simulink model "Measure_BH_curve1"  (R2014a)
settings: Solver=ode23tb  StartTime=0.0  StopTime=0.08  RelTol=1e-3
libraries: powerlib x9, simulink x1
settings Model: Creator=Administrator  LastModifiedBy=Administrator

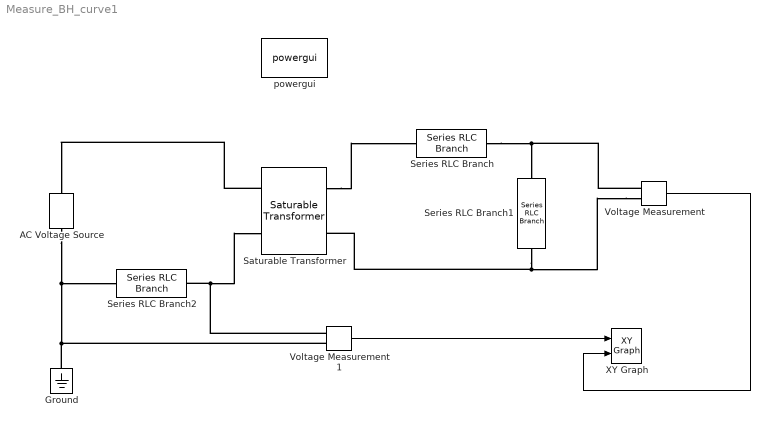
== system Measure_BH_curve1 ==
  AC Voltage Source : powerlib/Electrical Sources/AC Voltage Source  Amplitude=10e5*sqrt(2)  Phase=90  Frequency=50  SampleTime=0  Measurements=None
  Ground : powerlib/Elements/Ground  LConnTagsString=a
  Saturable Transformer : powerlib/Elements/Saturable Transformer  ThreeWindings=off  Hysteresis=off  DataFile='hysteresis.mat'  Measurements=None  UNITS=SI  NominalPower=[250e6 50]  Winding1=[7.35e+05 4.3218 0.55028]  Winding2=[3.15e+05 0.7938 0.10107]  Winding3=[3.15e+05 0.7938 0.10107]  Saturation=[0 0;0.0024001 1.2;1 1.52]  CoreLoss=1.0805e+06  MoreParameters=off  BreakLoop=off  DataType=off  InitialFlux=-1.07606886743008  TransfoNumber=1
  Series RLC Branch : powerlib/Elements/Series RLC Branch  LConnTagsString=__new0  RConnTagsString=__new0  BranchType=R  Resistance=400e3  Inductance=1e-3  SetiL0=off  InitialCurrent=0  Capacitance=1e-6  Setx0=off  InitialVoltage=0  Measurements=None
  Series RLC Branch1 : powerlib/Elements/Series RLC Branch  LConnTagsString=__new0  RConnTagsString=__new0  BranchType=C  Resistance=1  Inductance=1e-3  SetiL0=off  InitialCurrent=0  Capacitance=10e-6  Setx0=off  InitialVoltage=0  Measurements=None
  Series RLC Branch2 : powerlib/Elements/Series RLC Branch  LConnTagsString=__new0  RConnTagsString=__new0  BranchType=R  Resistance=1e3  Inductance=1e-3  SetiL0=off  InitialCurrent=0  Capacitance=1e-6  Setx0=off  InitialVoltage=0  Measurements=None
  Voltage Measurement : powerlib/Measurements/Voltage Measurement  PhasorSimulation=off  OutputType=Complex  PSBequivalent=0
  Voltage Measurement1 : powerlib/Measurements/Voltage Measurement  PhasorSimulation=off  OutputType=Complex  PSBequivalent=0
  XY Graph : simulink/Sinks/XY Graph  xmin=-6e3  xmax=6e3  ymin=-6e2  ymax=6e2  st=-1
  powergui : powerlib/powergui  Priority=1  SimulationMode=Discrete  SolverType=Tustin  SampleTime=50e-6  frequency=60  SPID=off  DisableSnubberDevices=off  DisableRonSwitches=off  DisableVfSwitches=off  SwTol=0  Interpol=off  DisplayEquations=off  Ts=0  methode=off  frequencyindice=50  Pbase=100e6  ErrMax=1e-4  Iterations=50  UnitsV=kV  UnitsW=MW  FunctionMessages=off  echomessages=off  HookPort=off  EnableUseOfTLC=off  x0status=blocks  RestoreLinks=warning  ResistiveCurrentMeasurement=off  Frange=[0:2:500]  Ylog=off  Xlog=on  ShowGrid=off  save=off  variable=ZData  structure=0  ZoomFFT=off  StartTime=0.0  cycles=1  DisplayStyle=1  fundamental=60  FreqAxis=off  MaxFrequency=1000  frequencyindicesteady=1  RmsSteady=1  display=off
  wires:
  Voltage Measurement/1 -> XY Graph/2
  Voltage Measurement1/1 -> XY Graph/1
  connections:
  Saturable Transformer/LConn1 -- AC Voltage Source/RConn1
  Saturable Transformer/RConn1 -- Series RLC Branch/LConn1
  Series RLC Branch/RConn1 -- Series RLC Branch1/LConn1 -- Voltage Measurement/LConn1
  Voltage Measurement/LConn2 -- Saturable Transformer/RConn2 -- Series RLC Branch1/RConn1
  AC Voltage Source/LConn1 -- Ground/LConn1 -- Voltage Measurement1/LConn2 -- Series RLC Branch2/LConn1
  Series RLC Branch2/RConn1 -- Saturable Transformer/LConn2 -- Voltage Measurement1/LConn1
